simulink model "CONTROL_CLASIC_MM_SCARA"  (R2025b)
settings: Solver=ode23t  StartTime=0.0  StopTime=10.0  RelTol=1e-3
libraries: SCR x5
settings Model: Creator=Michael  LastModifiedBy=Michael

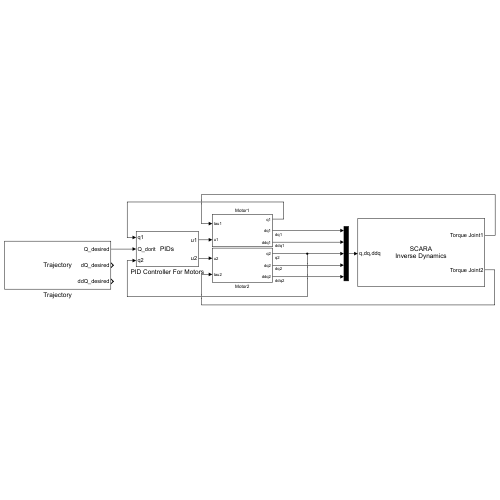
[thumbnail: Simulink's stored preview of the top-level diagram]
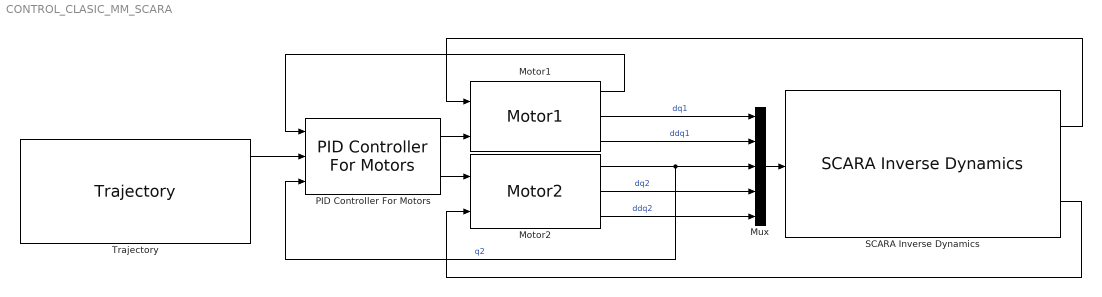
== system CONTROL_CLASIC_MM_SCARA ==
  Motor1 : SCR/Motor1  SystemSampleTime=-1  VariantActivationTime=update diagram  EmptyChoice=off  PassThrough=off  PassThroughVariantControl=(default)  EmptyChoiceVariantControl=(default)  AllowFlexibleInterface=on  Latency=0  AutoFrameSizeCalculation=off
  Motor2 : SCR/Motor2  SystemSampleTime=-1  VariantActivationTime=update diagram  EmptyChoice=off  PassThrough=off  PassThroughVariantControl=(default)  EmptyChoiceVariantControl=(default)  AllowFlexibleInterface=on  Latency=0  AutoFrameSizeCalculation=off
  Mux : Mux  Inputs=5
  PID Controller For Motors : SCR/PID Controller For Motors  SystemSampleTime=-1  VariantActivationTime=update diagram  EmptyChoice=off  PassThrough=off  PassThroughVariantControl=(default)  EmptyChoiceVariantControl=(default)  AllowFlexibleInterface=on  Latency=0  AutoFrameSizeCalculation=off
  SCARA Inverse Dynamics : SCR/SCARA Inverse Dynamics  SystemSampleTime=-1  VariantActivationTime=update diagram  EmptyChoice=off  PassThrough=off  PassThroughVariantControl=(default)  EmptyChoiceVariantControl=(default)  AllowFlexibleInterface=on  Latency=0  AutoFrameSizeCalculation=off
  Trajectory : SCR/Trajectory  SystemSampleTime=-1  VariantActivationTime=update diagram  EmptyChoice=off  PassThrough=off  PassThroughVariantControl=(default)  EmptyChoiceVariantControl=(default)  AllowFlexibleInterface=on  Latency=0  AutoFrameSizeCalculation=off
  wires:
  Trajectory/1 -> PID Controller For Motors/2
  Motor1/1 -> PID Controller For Motors/1
  Motor2/1 -> PID Controller For Motors/3, Mux/3  "q2"
  PID Controller For Motors/1 -> Motor1/2
  PID Controller For Motors/2 -> Motor2/1
  SCARA Inverse Dynamics/1 -> Motor1/1
  SCARA Inverse Dynamics/2 -> Motor2/2
  Mux/1 -> SCARA Inverse Dynamics/1
  Motor1/2 -> Mux/1  "dq1"
  Motor1/3 -> Mux/2  "ddq1"
  Motor2/2 -> Mux/4  "dq2"
  Motor2/3 -> Mux/5  "ddq2"
